simulink model "OPC_linea_transmision_observador"  (R2018a)
settings: Solver=VariableStepAuto  StartTime=0.0  StopTime=inf  RelTol=1e-3
InitFcn:
  | SimulinkInit_linea_transmision
values from neighbouring files (symbols this model uses):
  Ad = sysd.A    [SimulinkInit.m]
  Bd = sysd.B    [SimulinkInit.m]
  Cd = sysd.C    [SimulinkInit.m]
undefined symbols (not defined in the file or in its folder): C1o, C2o, C3o, C4o, F1, F2, F3, F4, H1, H2, H3, H4, K1U, K2U, K3U, K4U, T1, T2, T3, T4, tm
libraries: opclib x12, mpclib x1
settings Model: SimulationMode=accelerator  Creator=cmparedes  LastModifiedBy=MarioAndres

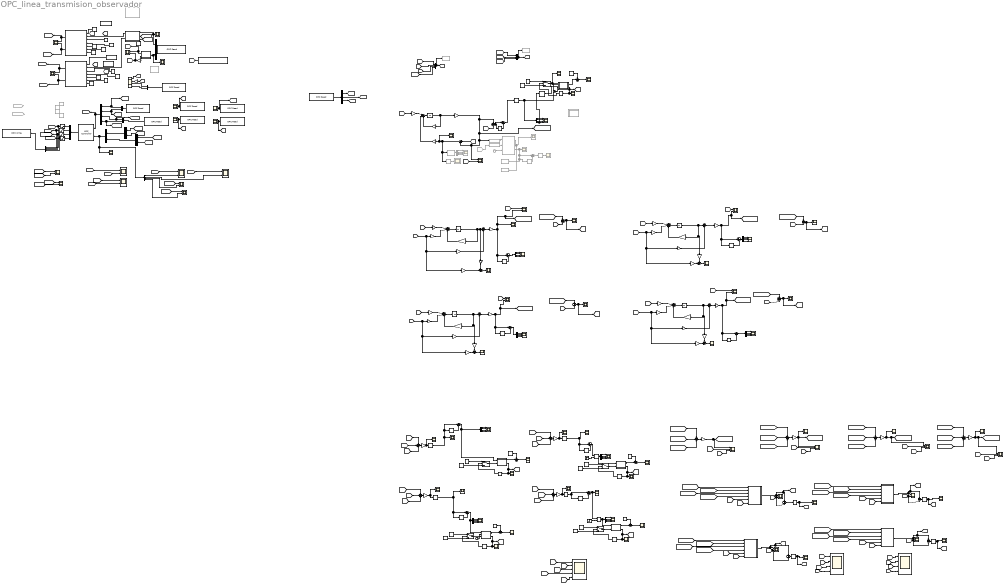
== system OPC_linea_transmision_observador ==
  note: CONTROL TERCIARIO
  note: Attack Quantification
  note: Attack Isolation I2
  note: Attack Isolation I1
  note: Attack Isolation Vsi
  note: Alarm I1
  note: Alarm I3
  note: Alarm I2
  note: Attack Detection
  note: Alarm V
  note: Attack Isolation I3
  Abs{,1..3,5..9} (9 alike) : Abs
  Abs4 : Abs  Commented=on
  Clock : Clock
  Clock1 : Clock  Commented=on
  Clock2 : Clock
  Constant : Constant  Value=2700
  Constant1 : Constant  Commented=on  Value=-13700
  Constant{7..8,10,12,14,22..23,27..28,32} (10 alike) : Constant
  Constant{9,11,21,24,31} (5 alike) : Constant  Value=0
  Constant13 : Constant  Value=500
  Constant15 : Constant  Value=1528
  Constant17 : Constant  Value=1154
  Constant18 : Constant  Value=1000
  Constant2 : Constant  Commented=on  Value=-400
  Constant3 : Constant  Commented=on  Value=5000
  Constant4 : Constant  Commented=on  Value=5000
  Constant5 : Constant  Commented=on  Value=8000
  Constant6 : Constant  Value=115400
  Delay : Delay  DelayLength=1
  Demux{,1..2,4} (4 alike) : Demux  Outputs=2
  Demux{3,5..14} (11 alike) : Demux
  Demux15 : Demux  Outputs=3
  Demux19 : Demux  Commented=on
  Derivative4 : Derivative  Commented=on  CoefficientInTFapproximation=0
  From27 : From  Commented=on  GotoTag=qbio_meas
  From28 : From  Commented=on  GotoTag=pbio_meas
  From60 : From  Commented=on  GotoTag=y_ma
  Gain1 : Gain  Gain=-1
  Gain17 : Gain
  Gain{22..29} (8 alike) : Gain  Gain=1/3
  LinearProg2 : MATLAB Function  TreatAsAtomicUnit=on  SystemSampleTime=1e-3
  LinearProg3 : MATLAB Function  TreatAsAtomicUnit=on  SystemSampleTime=1e-3
  MATLAB Funcionando sin Vload conectado despues del ataque : MATLAB Function  Commented=on  TreatAsAtomicUnit=on
  MATLAB Function : MATLAB Function  TreatAsAtomicUnit=on
  MATLAB Function1 : MATLAB Function  Commented=on  TreatAsAtomicUnit=on
  MATLAB Function12 : MATLAB Function  TreatAsAtomicUnit=on
  MATLAB Function13 : MATLAB Function  TreatAsAtomicUnit=on
  MATLAB Function17 : MATLAB Function  TreatAsAtomicUnit=on
  MATLAB Function18 : MATLAB Function  TreatAsAtomicUnit=on
  MATLAB Function2 : MATLAB Function  TreatAsAtomicUnit=on
  MATLAB Function3 : MATLAB Function  TreatAsAtomicUnit=on
  MATLAB Function34 : MATLAB Function  TreatAsAtomicUnit=on
  MATLAB Function36 : MATLAB Function  TreatAsAtomicUnit=on
  MATLAB Function38 : MATLAB Function  TreatAsAtomicUnit=on
  MATLAB Function39 : MATLAB Function  TreatAsAtomicUnit=on
  MATLAB Function7 : MATLAB Function  Commented=on  TreatAsAtomicUnit=on
  MATLAB Function8 : MATLAB Function  Commented=on  TreatAsAtomicUnit=on
  MPC Controller : mpclib/MPC Controller  SCDEnableBlockLinearizationSpecification=on  mpcobj=mpcobj  is_multiple=0  enable_value=0  return_u0=off  updateMPCinCallerWorkspace=on  ref_from_ws=off  ref_signal_name=[]  ref_preview=off  md_from_ws=off  md_signal_name=[]  md_preview=off  from_project=off  project_file=MPCtask.mat  md_inport=off  mv_inport=off  cost_outport=off  return_sequence=off  return_qpstatus=off  return_state=off  state_inport=off  lims_inport=off  cc_inport=off  ywt_inport=off  is_designfromscratch=0  uwt_inport=off  duwt_inport=off  rhoeps_inport=off  uref_inport=off  n_ts=0.1  n_p=100  n_mv=4  n_md=0  n_ud=0  n_mo=4  n_uo=0  BlockDataType=double  SampleTimeInherited=off  switch_inport=off
  Memory{,1..13} (14 alike) : Memory
  Memory14 : Memory  Commented=on
  Mux : Mux
  Mux3 : Mux  Inputs=2
  Mux4 : Mux
  Mux5 : Mux  Inputs=2
  Mux6 : Mux  Inputs=2
  Mux7 : Mux  Inputs=3
  Mux8 : Mux
  OPC Configuration : opclib/OPC Configuration  opcServers=localhost/Kepware.KEPServerEX.V6/10  errMissingItems=Error  errReadWrite=Warn  errShutdown=Error  errRTViolation=Warn  rtEnable=on  speedup=1  showLatency=off  beingUsed=on
      settings: SourceProductName=OPC Toolbox  SourceProductBaseCode=OT
  OPC Read : opclib/OPC Read  serverHost=localhost  serverID=Kepware.KEPServerEX.V6  itemIDs=Carga_Reno_Channel.Carga.Group1.SOC, Carga_Reno_Channel.Carga.Group1.Lref  readMode=Synchronous (cache)  dataType=double  updateRate=0.1  showQual=off  showTS=off  tsMode=Seconds since start
      settings: SourceProductName=OPC Toolbox  SourceProductBaseCode=OT
  OPC Read1 : opclib/OPC Read  serverHost=localhost  serverID=Kepware.KEPServerEX.V6  itemIDs=Carga_Reno_Channel.Carga.Group1.Vload  readMode=Synchronous (cache)  dataType=double  updateRate=0.1  showQual=off  showTS=off  tsMode=Seconds since start
      settings: SourceProductName=OPC Toolbox  SourceProductBaseCode=OT
  OPC Read2 : opclib/OPC Read  serverHost=localhost  serverID=Kepware.KEPServerEX.V6  itemIDs=Bio_Channel.Bio.Group1.Ibio  readMode=Synchronous (cache)  dataType=double  updateRate=0.1  showQual=off  showTS=off  tsMode=Seconds since start
      settings: SourceProductName=OPC Toolbox  SourceProductBaseCode=OT
  OPC Read3 : opclib/OPC Read  serverHost=localhost  serverID=Kepware.KEPServerEX.V6  itemIDs=Diesel_Channel.Diesel.Group1.Idiesel  readMode=Synchronous (cache)  dataType=double  updateRate=0.1  showQual=off  showTS=off  tsMode=Seconds since start
      settings: SourceProductName=OPC Toolbox  SourceProductBaseCode=OT
  OPC Read4 : opclib/OPC Read  serverHost=localhost  serverID=Kepware.KEPServerEX.V6  itemIDs=Carga_Reno_Channel.Carga.Group1.Pm, Carga_Reno_Channel.Carga.Group1.Qm  readMode=Synchronous (cache)  dataType=double  updateRate=0.1  showQual=off  showTS=off  tsMode=Seconds since start
      settings: SourceProductName=OPC Toolbox  SourceProductBaseCode=OT
  OPC Read5 : opclib/OPC Read  serverHost=localhost  serverID=Kepware.KEPServerEX.V6  itemIDs=Carga_Reno_Channel.Carga.Group1.KB  readMode=Synchronous (cache)  dataType=double  updateRate=0.1  showQual=off  showTS=off  tsMode=Seconds since start
      settings: SourceProductName=OPC Toolbox  SourceProductBaseCode=OT
  OPC Read6 : opclib/OPC Read  serverHost=localhost  serverID=Kepware.KEPServerEX.V6  itemIDs=Carga_Reno_Channel.Carga.Group1.Ipv  readMode=Synchronous (cache)  dataType=double  updateRate=0.1  showQual=off  showTS=off  tsMode=Seconds since start
      settings: SourceProductName=OPC Toolbox  SourceProductBaseCode=OT
  OPC Read7 : opclib/OPC Read  serverHost=localhost  serverID=Kepware.KEPServerEX.V6  itemIDs=Bio_Channel.Bio.Group1.Pm, Bio_Channel.Bio.Group1.Qm  readMode=Synchronous (cache)  dataType=double  updateRate=0.1  showQual=off  showTS=off  tsMode=Seconds since start
      settings: SourceProductName=OPC Toolbox  SourceProductBaseCode=OT
  OPC Read8 : opclib/OPC Read  serverHost=localhost  serverID=Kepware.KEPServerEX.V6  itemIDs=Carga_Reno_Channel.Carga.Group1.Po_reno, Carga_Reno_Channel.Carga.Group1.Qo_reno  readMode=Synchronous (cache)  dataType=double  updateRate=0.1  showQual=off  showTS=off  tsMode=Seconds since start
      settings: SourceProductName=OPC Toolbox  SourceProductBaseCode=OT
  OPC Read9 : opclib/OPC Read  serverHost=localhost  serverID=Kepware.KEPServerEX.V6  itemIDs=Bio_Channel.Bio.Group1.DuC, Carga_Reno_Channel.Carga.Group1.DuC_reno, Diesel_Channel.Diesel.Group1.DieselDutyC  readMode=Synchronous (cache)  dataType=double  updateRate=0.1  showQual=off  showTS=off  tsMode=Seconds since start
      settings: SourceProductName=OPC Toolbox  SourceProductBaseCode=OT
  OPC Write : opclib/OPC Write  serverHost=localhost  serverID=Kepware.KEPServerEX.V6  itemIDs=Bio_Channel.Bio.Group1.Pref, Bio_Channel.Bio.Group1.Qref, Carga_Reno_Channel.Carga.Group1.Pi_reno, Carga_Reno_Channel.Carga.Group1.Qi_reno  writeMode=Synchronous  updateRate=0
      settings: SourceProductName=OPC Toolbox  SourceProductBaseCode=OT
  Pbmax : Constant  Value=1000
  Pbmax1 : Constant  Value=1000
  Pdmax : Constant  Value=1200
  Pdmax1 : Constant  Value=800
  Product2 : Product
  Product4 : Product
  Saturation : Saturate  UpperLimit=12000  LowerLimit=-10000
  Saturation1 : Saturate  UpperLimit=12000  LowerLimit=-10000
  Saturation2 : Saturate  UpperLimit=14000  LowerLimit=-10000
  Saturation3 : Saturate  UpperLimit=10000  LowerLimit=-10000
  Scope{,2..3,7..9,25,30..32,34,41..49,51,55..57,61,64..73,75,110,112,114,118,120..121,135} (43 alike) : Scope
  Scope{1,5..6,10..18,52..53,58,86..89,109} (20 alike) : Scope  NumInputPorts=2
  Scope{59..60,62,138} (4 alike) : Scope  NumInputPorts=3
  Scope{19,36,50,139} (4 alike) : Scope  Commented=on
  Scope{4,33,63,76..83,85} (12 alike) : Scope  NumInputPorts=4
  Scope54 : Scope  Commented=on  NumInputPorts=4
  Scope84 : Scope  NumInputPorts=5
  Signal Specification : SignalSpecification  Commented=on  Dimensions=4
  Signal Specification1 : SignalSpecification  Commented=on  Dimensions=4
  Step13 : Step  Time=0.1  SampleTime=0
  Step14 : Step  Time=0.1  SampleTime=0
  Sum{10,22,38,74} (4 alike) : Sum  Inputs=|++
  Sum{16,18,27,33,42,67,70,72..73} (9 alike) : Sum  Inputs=+-
  Sum{17,20,24..26,30,36..37,39..40} (10 alike) : Sum  Inputs=|+-
  Sum{19,31..32,71} (4 alike) : Sum  Inputs=-+|
  Sum{21,23,49,75..76} (5 alike) : Sum  Inputs=|+++  SampleTime=tm
  Sum{28..29,34..35,53} (5 alike) : Sum  Inputs=+-|
  Sum41 : Sum  Commented=on  Inputs=|+-
  Sum{58..61,77..80} (8 alike) : Sum  Inputs=+++
  Switch{,1..4} (5 alike) : Switch  Criteria=u2 > Threshold
  To Workspace : ToWorkspace  Commented=on  VariableName=det1  SampleTime=1e-4
  To Workspace1 : ToWorkspace  Commented=on  VariableName=norm1  SampleTime=1e-4
  To Workspace2 : ToWorkspace  Commented=on  VariableName=y_ma  SampleTime=1e-4
  To Workspace3 : ToWorkspace  Commented=on  VariableName=u_fs  SampleTime=1e-4
  Unit Delay{1..2,6..7,10} (5 alike) : UnitDelay  SampleTime=tm
  adis1 : Gain  Gain=F3  Multiplication=Matrix(K*u) (u vector)  SampleTime=tm
  adis10 : Gain  Gain=Ld'  Multiplication=Matrix(K*u) (u vector)  SampleTime=tm
  adis11 : Gain  Gain=F1  Multiplication=Matrix(K*u) (u vector)  SampleTime=tm
  adis12 : Gain  Gain=F2  Multiplication=Matrix(K*u) (u vector)  SampleTime=tm
  adis2 : Gain  Gain=F4  Multiplication=Matrix(K*u) (u vector)  SampleTime=tm
  adis7 : Gain  Gain=Ad  Multiplication=Matrix(K*u) (u vector)  SampleTime=tm
  bdis1 : Gain  Gain=T3*Bd  Multiplication=Matrix(K*u) (u vector)  SampleTime=tm
  bdis10 : Gain  Gain=T2*Bd  Multiplication=Matrix(K*u) (u vector)  SampleTime=tm
  bdis11 : Gain  Gain=K2U  Multiplication=Matrix(K*u) (u vector)  SampleTime=tm
  bdis12 : Gain  Gain=H2  Multiplication=Matrix(K*u) (u vector)  SampleTime=tm
  bdis13 : Gain  Gain=eye(1)-C2o*H2  Multiplication=Matrix(K*u) (u vector)  SampleTime=tm
  bdis14 : Gain  Gain=eye(1)-C1o*H1  Multiplication=Matrix(K*u) (u vector)  SampleTime=tm
  bdis15 : Gain  Gain=C1o  Multiplication=Matrix(K*u) (u vector)  SampleTime=tm
  bdis16 : Gain  Gain=C2o  Multiplication=Matrix(K*u) (u vector)  SampleTime=tm
  bdis17 : Gain  Gain=T4*Bd  Multiplication=Matrix(K*u) (u vector)  SampleTime=tm
  bdis18 : Gain  Gain=K4U  Multiplication=Matrix(K*u) (u vector)  SampleTime=tm
  bdis19 : Gain  Gain=H4  Multiplication=Matrix(K*u) (u vector)  SampleTime=tm
  bdis2 : Gain  Gain=K3U  Multiplication=Matrix(K*u) (u vector)  SampleTime=tm
  bdis20 : Gain  Gain=eye(1)-C4o*H4  Multiplication=Matrix(K*u) (u vector)  SampleTime=tm
  bdis21 : Gain  Gain=C4o  Multiplication=Matrix(K*u) (u vector)  SampleTime=tm
  bdis3 : Gain  Gain=H3  Multiplication=Matrix(K*u) (u vector)  SampleTime=tm
  bdis4 : Gain  Gain=eye(1)-C3o*H3  Multiplication=Matrix(K*u) (u vector)  SampleTime=tm
  bdis5 : Gain  Gain=Bd  Multiplication=Matrix(K*u) (u vector)  SampleTime=tm
  bdis6 : Gain  Gain=C3o  Multiplication=Matrix(K*u) (u vector)  SampleTime=tm
  bdis7 : Gain  Gain=T1*Bd  Multiplication=Matrix(K*u) (u vector)  SampleTime=tm
  bdis8 : Gain  Gain=K1U  Multiplication=Matrix(K*u) (u vector)  SampleTime=tm
  bdis9 : Gain  Gain=H1  Multiplication=Matrix(K*u) (u vector)  SampleTime=tm
  cdis{1..5} (5 alike) : Gain  Gain=Cd  Multiplication=Matrix(K*u) (u vector)  SampleTime=tm
  kbP : Constant
  kbQ : Constant
  kdP : Constant
  kdQ : Constant
  wires:
  LinearProg2/1(Pbo) -> [Pbio], Scope16/1
  LinearProg2/2(Pdo) -> [Pdiesel], Scope16/2
  Pdmax1/1 -> LinearProg3/5(QdMax)
  kdP/1 -> LinearProg2/4(kd)
  LinearProg3/2(Qdo) -> Scope15/2, [Qdiesel]
  MATLAB Function2/2(MaxQ) -> LinearProg3/2(Q_e_alt)
  LinearProg3/1(Qbo) -> [Qbio], Scope15/1
  MATLAB Function2/1(MaxP) -> LinearProg2/2(P_e_alt)
  kdQ/1 -> LinearProg3/4(kd)
  Gain17/1 -> Scope1/2, [Q_load]
  OPC Read/1 -> Demux1/1
  Demux1/1 -> MATLAB Function2/1(SOC), Scope2/1
  MATLAB Function/2(Qref) -> Gain17/1
  MATLAB Function/1(Pref) -> Scope1/1, [P_load]
  OPC Read4/1 -> Demux2/1
  Demux2/1 -> Scope4/3
  Demux2/2 -> Scope4/4
  [P_load] -> Scope4/1
  Demux1/2 -> Scope/1, MATLAB Function/1(Lref)
  Gain1/1 -> Scope4/2
  [Q_load] -> Gain1/1
  OPC Read5/1 -> [Kb]
  Constant15/1 -> LinearProg2/1(P_load)
  Pdmax/1 -> LinearProg2/5(PdMax)
  Pbmax/1 -> LinearProg2/6(PbMax)
  Constant18/1 -> LinearProg2/7(P_e_alt_min)
  Pbmax1/1 -> LinearProg3/6(QbMax)
  Constant13/1 -> LinearProg3/7(Q_e_alt_min)
  Demux/2 -> Mux4/2, [Qo_bio]
  Demux3/4 -> Saturation3/1
  MPC Controller/1 -> Demux3/1
  Demux3/3 -> Saturation2/1
  Mux6/1 -> Mux3/2
  Demux4/2 -> [Qo_diesel], Mux4/4
  Demux3/1 -> Saturation/1
  Demux3/2 -> Saturation1/1
  Mux4/1 -> [Paparente], MPC Controller/1
  Demux/1 -> Mux4/1, [Po_bio]
  Mux5/1 -> Mux3/1
  [Pbio] -> Mux5/1
  [Qbio] -> Mux5/2
  [Pdiesel] -> Mux6/1
  [Qdiesel] -> Mux6/2
  [Qo_diesel] -> Scope17/1
  [Qi_bio] -> Scope5/2
  [Po_diesel] -> Scope18/1
  [Pi_Diesel] -> Scope18/2
  [Qi_diesel] -> Scope17/2
  [Pi_bio] -> Scope6/2
  [Qo_bio] -> Scope5/1
  [Po_bio] -> Scope6/1
  OPC Read1/1 -> [V_vsi], Scope3/1
  OPC Read2/1 -> [I1], Scope7/1
  OPC Read3/1 -> [I3], Scope8/1
  OPC Read6/1 -> [I2], Scope9/1
  OPC Read7/1 -> Demux/1
  OPC Read8/1 -> Demux4/1
  Demux4/1 -> [Po_diesel], Mux4/3
  kbP/1 -> LinearProg2/3(kb)
  Constant6/1 -> LinearProg3/1(Q_load)
  [Qo_diesel] -> MATLAB Function2/2(q)
  [Po_diesel] -> MATLAB Function2/3(p)
  kbQ/1 -> LinearProg3/3(kb)
  Saturation/1 -> Mux/1, [Pi_bio]
  Saturation1/1 -> Mux/2, [Qi_bio]
  Saturation2/1 -> Mux/3, [Pi_Diesel]
  Saturation3/1 -> Mux/4, [Qi_diesel]
  Mux/1 -> OPC Write/1
  [Po_diesel] -> Scope11/1
  [Qo_bio] -> Scope12/1
  [Po_bio] -> Scope13/1
  [Qo_diesel] -> Scope10/1
  Mux3/1 -> Demux6/1, Scope32/1, MPC Controller/2
  Demux6/1 -> Scope13/2
  Demux6/2 -> Scope12/2
  Demux6/3 -> Scope11/2
  Demux6/4 -> Scope10/2
  [e2] -> Scope63/2
  Step14/1 -> Product4/2
  Product4/1 -> MATLAB Function18/1(dr), Demux13/1
  Sum77/1 -> Gain22/1
  Clock/1 -> MATLAB Function12/4(t)
  [y_ma] -> Sum70/2
  bdis3/1 -> Sum38/2
  bdis16/1 -> Sum32/1
  [I3] -> Mux8/3
  Sum24/1 -> Demux11/1, MATLAB Function13/1(dr)
  [y_ma] -> Sum17/1
  [x_hat_uio11] -> Sum58/1
  Clock2/1 -> MATLAB Function13/3(t)
  [x_hat_uio21] -> Sum67/1
  Switch/1 -> MATLAB Function36/2(ban)
  Sum35/1 -> Scope51/1
  [y_ma] -> Scope60/3
  Sum10/1 -> cdis1/1
  Demux12/1 -> Scope82/1
  Product2/1 -> MATLAB Function17/1(dr), Demux12/1
  Sum32/1 -> Scope66/1
  Signal Specification1/1 -> MATLAB Function8/2(y_m)
  Sum41/1 -> Abs4/1
  Sum16/1 -> Abs6/1
  Demux5/4 -> Scope77/4
  Sum38/1 -> cdis3/1
  [x_hat_uio1] -> MATLAB Function3/1(x_hat1)
  Constant9/1 -> Switch1/1
  [ca1] -> Scope85/1
  Mux7/1 -> To Workspace3/1, [u_fs]
  Sum73/1 -> [druo3], Scope44/1
  [ca4] -> Scope85/4
  [x_hat] -> Scope60/2
  [V_vsi] -> Mux8/4
  [x_hat_uio11] -> Sum60/1
  [rol] -> MATLAB Function34/6(rol)
  [I2] -> bdis14/1, bdis9/1, bdis8/1
  Abs7/1 -> [e2], Scope70/1
  [x_hat_uio2] -> MATLAB Function34/2(x_hat2)
  Demux9/2 -> Scope79/2
  [y_ma] -> Scope59/3
  Abs8/1 -> [e4], Scope71/1
  [I1] -> Mux8/1
  [y_ma] -> Scope62/3
  [y_ma] -> Scope138/3
  [x_hat] -> Scope138/2
  [a3] -> Sum42/2, Scope58/2
  Switch4/1 -> MATLAB Function13/2(ban)
  Sum61/1 -> Gain27/1
  Sum42/1 -> Abs9/1
  Demux9/4 -> Scope79/4
  Gain24/1 -> Abs1/1, Scope114/1
  Delay/1 -> MATLAB Function12/3(dr1)
  Demux7/3 -> Scope76/3
  Memory6/1 -> Switch2/2
  [ca2] -> Scope85/2
  Sum20/1 -> Demux10/1, MATLAB Function36/1(dr)
  Step13/1 -> Product2/2
  [ruo3] -> Scope84/4
  bdis1/1 -> Sum49/1
  Memory2/1 -> Sum24/2
  Abs1/1 -> Memory2/1, Sum24/1, Scope31/1
  Gain29/1 -> Scope59/1, Scope41/1, [x_hat_uio2]
  Demux13/1 -> Scope83/1
  Constant27/1 -> Switch3/3
  MATLAB Function3/1(v1) -> [ca4], Sum27/1, Scope52/1
  Sum18/1 -> Abs7/1
  Gain22/1 -> Abs/1, Scope110/1
  Abs6/1 -> [e1], Scope64/1
  [e1] -> Scope63/1
  Sum60/1 -> Gain26/1
  [x_hat] -> Scope59/2
  [a4] -> Sum27/2, Scope52/2
  [x_hat_uio12] -> Sum58/2
  Gain27/1 -> Scope135/1, Scope62/1, [x_hat_uio4]
  Sum29/1 -> Scope55/1
  Demux8/1 -> Scope78/1
  [a2] -> Sum18/2, Scope53/2
  [x_hat_uio3] -> MATLAB Function3/3(x_hat3)
  Abs9/1 -> [e3], Scope73/1
  [rol] -> MATLAB Function3/6(rol)
  [ruo4] -> MATLAB Function3/5(ruo1)
  Constant31/1 -> Switch4/1
  [x_hat_uio12] -> Sum59/2
  [x_hat_uio3] -> MATLAB Function34/3(x_hat3)
  Demux9/3 -> Scope79/3
  Gain28/1 -> Scope138/1, [x_hat_uio1]
  Sum37/1 -> Demux5/1
  Gain26/1 -> Scope42/1, Scope60/1, [x_hat_uio3]
  [x_hat] -> Scope62/2
  [x_hat_uio21] -> Sum59/1
  [x_hat_uio13] -> Sum59/3
  [x_hat_uio21] -> Sum60/3
  [x_hat_uio3] -> MATLAB Function38/3(x_hat3)
  [u3] -> Mux7/3
  Memory9/1 -> Switch4/2
  [y_ma] -> Scope88/1
  MATLAB Function39/1(v1) -> [ca3], Sum42/1, Scope58/1
  MATLAB Function8/1(rol) -> To Workspace/1, Scope19/1
  [x_hat_uio4] -> MATLAB Function3/4(x_hat4)
  [ruo2] -> MATLAB Function34/5(ruo1)
  Sum39/1 -> Demux8/1
  [x_hat_uio11] -> Sum61/1
  Demux9/1 -> Scope79/1
  [e4] -> Scope63/4
  bdis4/1 -> Sum71/2
  [x_hat_uio4] -> MATLAB Function34/4(x_hat4)
  [druo2] -> Sum78/1
  [ruo2] -> Scope84/3
  Sum36/1 -> Demux7/1
  [ruo1] -> MATLAB Function38/5(ruo1)
  [x_hat_uio1] -> MATLAB Function39/1(x_hat1)
  [x_hat_uio13] -> Sum58/3
  Constant32/1 -> Switch4/3
  Demux13/3 -> Scope83/3
  [x_hat_uio4] -> MATLAB Function39/4(x_hat4)
  bdis18/1 -> Sum76/2
  Demux5/2 -> Scope77/2
  Demux13/4 -> Scope83/4
  cdis3/1 -> Memory12/1, Sum39/1, Scope88/2, [x_hat_uio13]
  [u_fs] -> bdis5/1
  Abs4/1 -> Scope36/1
  Memory14/1 -> Sum41/2
  bdis11/1 -> Sum23/2
  [rol] -> MATLAB Function39/6(rol)
  [druo1] -> Sum77/1
  Abs5/1 -> Demux14/1, MATLAB Function12/1(dr)
  Demux14/2 -> Scope33/2
  Demux14/3 -> Scope33/3
  Demux12/3 -> Scope82/3
  Constant22/1 -> Switch2/3
  Demux12/4 -> Scope82/4
  Demux12/2 -> Scope82/2
  Demux11/3 -> Scope81/3
  [x_hat_uio2] -> MATLAB Function38/2(x_hat2)
  Demux11/1 -> Scope81/1
  Demux10/3 -> Scope80/3
  Demux10/4 -> Scope80/4
  Demux10/1 -> Scope80/1
  [x_hat_uio2] -> MATLAB Function3/2(x_hat2)
  Abs2/1 -> Memory3/1, Sum25/1, Scope34/1
  Demux14/1 -> Scope33/1
  Sum33/1 -> Sum30/1, Memory7/1
  Demux14/4 -> Delay/1, Scope33/4
  Sum25/1 -> Product2/1
  Sum17/1 -> Derivative4/1, MATLAB Function7/1(r), Scope48/1, adis10/1
  Demux8/3 -> Scope78/3
  Demux8/2 -> Scope78/2
  [x_hat_uio4] -> MATLAB Function38/4(x_hat4)
  Demux7/2 -> Scope76/2
  Demux5/3 -> Scope77/3
  [x_hat_uio3] -> MATLAB Function39/3(x_hat3)
  [x_hat_uio11] -> Sum70/1
  Switch1/1 -> MATLAB Function17/2(ban)
  Demux5/1 -> Scope77/1
  [u1] -> Mux7/1
  Demux11/2 -> Scope81/2
  Abs/1 -> Memory/1, Sum20/1, Scope25/1
  Memory13/1 -> Sum40/2
  Memory7/1 -> Sum30/2
  Memory11/1 -> Sum37/2
  [x_hat_uio1] -> MATLAB Function38/1(x_hat1)
  [a1] -> Sum16/2, Scope109/2
  Memory10/1 -> Sum36/2
  Sum79/1 -> Gain24/1
  Constant28/1 -> Sum35/1
  Sum75/1 -> Unit Delay6/1
  Unit Delay2/1 -> bdis21/1, adis2/1, Sum74/1
  bdis2/1 -> Sum49/2
  Demux8/4 -> Scope78/4
  Sum30/1 -> Abs5/1
  MATLAB Function12/1(r) -> Sum34/2
  Sum34/1 -> Scope68/1
  [u2] -> Mux7/2
  [ruo3] -> MATLAB Function39/5(ruo1)
  Memory8/1 -> Switch3/2
  MATLAB Function34/1(v1) -> [ca2], Sum18/1, Scope53/1
  Switch3/1 -> Scope75/1, MATLAB Function12/2(ban)
  Constant23/1 -> Sum34/1
  MATLAB Function18/1(r) -> Sum29/2
  Memory12/1 -> Sum39/2
  Constant21/1 -> Switch2/1
  [x_hat_uio2] -> MATLAB Function39/2(x_hat2)
  [druo3] -> Sum77/3
  Memory/1 -> Sum20/2
  MATLAB Function17/2(c) -> [ruo2], Scope49/1, Memory5/1
  MATLAB Function13/1(r) -> Sum35/2
  [x_hat_uio1] -> MATLAB Function34/1(x_hat1)
  MATLAB Function13/2(c) -> [ruo3], Scope57/1, Memory9/1
  [I1] -> bdis20/1, bdis19/1, bdis18/1
  Constant11/1 -> Switch/1
  [druo2] -> Sum77/2
  Constant10/1 -> Switch1/3
  Constant8/1 -> Sum28/1
  Memory4/1 -> Sum26/2
  Memory3/1 -> Sum25/2
  Constant7/1 -> Sum53/1
  MATLAB Function12/2(c) -> [rol], Scope69/1, Memory8/1
  [ca3] -> Scope85/3
  Memory1/1 -> Switch/2
  Sum53/1 -> Scope120/1
  bdis6/1 -> Sum71/1
  MATLAB Function36/2(c) -> [ruo1], Scope121/1, Memory1/1
  [y_ma] -> Sum33/2
  Sum78/1 -> Gain23/1
  MATLAB Function38/1(v1) -> [ca1], Sum16/1, Scope109/1
  Sum72/1 -> [druo2], Scope43/1
  MATLAB Function17/1(r) -> Sum28/2
  Constant12/1 -> Sum29/1
  [x_hat_uio21] -> Sum61/2
  [x_hat_uio13] -> Sum60/2
  [ruo4] -> Scope84/5
  Gain25/1 -> Scope118/1, Abs3/1
  Sum26/1 -> Product4/1, Scope46/1
  Constant24/1 -> Switch3/1
  Demux7/4 -> Scope76/4
  Gain23/1 -> Abs2/1, Scope112/1
  MATLAB Function18/2(c) -> [ruo4], Scope56/1, Memory6/1
  [rol] -> MATLAB Function38/6(rol)
  [druo2] -> Sum80/2
  Sum80/1 -> Gain25/1
  [druo1] -> Sum79/2
  adis7/1 -> Sum75/3
  [x_hat_uio12] -> Sum61/3
  [druo4] -> Sum78/3
  [druo3] -> Sum78/2
  [x_hat_uio13] -> Sum73/1
  [y_ma] -> Sum72/2
  Sum67/1 -> [druo4], Scope45/1
  [x_hat_uio12] -> Sum72/1
  [y_ma] -> Sum67/2
  bdis8/1 -> Sum21/2
  Demux19/1 -> Scope54/1
  Sum58/1 -> Gain28/1
  Demux13/2 -> Scope83/2
  Sum70/1 -> [druo1], Scope30/1
  Sum28/1 -> Scope47/1
  Sum27/1 -> Abs8/1
  [e3] -> Scope63/3
  cdis1/1 -> Memory10/1, Sum36/1, [x_hat_uio11], Scope86/2, Scope61/1
  [druo3] -> Sum79/1
  Constant14/1 -> Switch/3
  [druo1] -> Sum80/3
  Switch2/1 -> MATLAB Function18/2(ban)
  [druo4] -> Sum80/1
  cdis2/1 -> Memory11/1, Sum37/1, Scope87/2, [x_hat_uio12]
  Demux10/2 -> Scope80/2
  Sum71/1 -> Scope67/1
  Memory5/1 -> Switch1/2
  Sum74/1 -> cdis5/1
  Sum31/1 -> Scope65/1
  bdis19/1 -> Sum74/2
  Sum22/1 -> cdis2/1
  [y_ma] -> Scope87/1
  adis2/1 -> Sum76/3
  [u_fs] -> bdis1/1
  bdis20/1 -> Sum19/2
  Sum19/1 -> Scope72/1
  cdis4/1 -> Sum33/1, [x_hat], Signal Specification/1, Scope14/1, Sum17/2
  bdis7/1 -> Sum21/1
  [druo4] -> Sum79/3
  Sum23/1 -> Unit Delay10/1
  bdis17/1 -> Sum76/1
  adis1/1 -> Sum49/3
  Demux7/1 -> Scope76/1
  [I3] -> bdis13/1, bdis12/1, bdis11/1
  Sum21/1 -> Unit Delay7/1
  adis10/1 -> Sum75/2
  Sum40/1 -> Demux9/1
  Demux11/4 -> Scope81/4
  bdis14/1 -> Sum31/2
  Abs3/1 -> Memory4/1, Sum26/1
  Unit Delay1/1 -> bdis6/1, adis1/1, Sum38/1
  Sum76/1 -> Unit Delay2/1
  adis11/1 -> Sum21/3
  Demux19/2 -> Scope54/2
  Unit Delay6/1 -> cdis4/1, adis7/1
  [u_fs] -> bdis10/1
  adis12/1 -> Sum23/3
  bdis10/1 -> Sum23/1
  MATLAB Function36/1(r) -> Sum53/2
  [u_fs] -> bdis7/1
  Demux19/3 -> Scope54/3
  Sum59/1 -> Gain29/1
  [y_ma] -> Scope14/2
  Demux19/4 -> Scope54/4
  [y_ma] -> Scope86/1
  Clock1/1 -> MATLAB Function8/3(tiempo)
  From60/1 -> Signal Specification1/1
  bdis13/1 -> Sum32/2
  cdis5/1 -> Memory13/1, Sum40/1, [x_hat_uio21], Scope89/2
  Derivative4/1 -> Scope139/1
  Mux8/1 -> To Workspace2/1, [y_ma]
  Sum49/1 -> Unit Delay1/1
  bdis9/1 -> Sum10/2
  [rol] -> Scope84/1
  Unit Delay7/1 -> adis11/1, bdis15/1, Sum10/1
  [I2] -> Mux8/2
  bdis12/1 -> Sum22/2
  bdis5/1 -> Sum75/1
  [y_ma] -> Scope89/1
  MATLAB Function8/2(norm_rd) -> Sum41/1, Memory14/1, To Workspace1/1, Scope50/1
  bdis21/1 -> Sum19/1
  [u_fs] -> bdis17/1
  MATLAB Function7/1(y) -> Demux19/1
  bdis15/1 -> Sum31/1
  [ruo1] -> Scope84/2
  Unit Delay10/1 -> bdis16/1, adis12/1, Sum22/1
  [y_ma] -> Sum73/2
  [V_vsi] -> bdis4/1, bdis3/1, bdis2/1
  Signal Specification/1 -> MATLAB Function8/1(y_hat)
  OPC Read9/1 -> Demux15/1
  Demux15/1 -> [u1]
  Demux15/2 -> [u2]
  Demux15/3 -> [u3]

== matlab function OPC_linea_transmision_observador/MATLAB Function ==
  data: Lref input; Pref output; Qref output
function [Pref,Qref] = fcn(Lref)

Pref = 1000;
Qref = 1000;%sqrt(Lref^2 - Pref^2);

== matlab function OPC_linea_transmision_observador/MATLAB Function3 ==
  data: x_hat1 input; v1 output; x_hat2 input; x_hat3 input; x_hat4 input; ruo1 input; rol input
function v1 = fcn(x_hat1,x_hat2,x_hat3,x_hat4,ruo1,rol)

% yol=[u1 ; u2];
% ym=[ym1 ; ym2];
%  C1=[zeros(1,10) 1];
 C1=[0 0 0 1];
 v11=C1*(x_hat4-x_hat1)*ruo1*rol;
 v12=C1*(x_hat4-x_hat2)*ruo1*rol;
 v13=C1*(x_hat4-x_hat3)*ruo1*rol;
 
 v1=-(v11+v12+v13);

== matlab function OPC_linea_transmision_observador/LinearProg2 ==
  data: P_load input; Pbo output; P_e_alt input; kb input; kd input; PdMax input; PbMax input; Pdo output; P_e_alt_min input
function [Pbo, Pdo] = fcn(P_load, P_e_alt, kb, kd, PdMax, PbMax, P_e_alt_min)

% P_load es la potencia que se requiere en la carga.

% P_e_alt es la potencia estimada de generacion de las energias
% alternativas

% kb y kd son los pesos de las funcion de costo.

% las salidas son las potencias optimas para bio y diesel

Pb=0;
Pd=0;

D_P_e_alt = P_e_alt - P_e_alt_min; % superaavit de energia alternativa.

flagDelt = 0;

if(D_P_e_alt >= P_load)
    flagDelt = 1;
end
   

if(flagDelt==0)
    P_trad = P_load - D_P_e_alt;
    % flag: variable que indica si tiene sentido evaluar los
    % if's que se encuentran mas adelante. es decir, si flag = 0 
    % despues del primer if entonces NO se le esta pidiendo al sistema
    % mas potencia de la que puede generar y portanto el problema de 
    % optimizacion lineal tiene sentido.
    % entonces 
    flag=0;

    if(P_trad>PdMax+PbMax)
        Pd=PdMax;
        Pb=PbMax;
        flag=1;
    end

    % si ambas energias tienen el mismo factor de costo.
    if(kd==kb && flag==0)
        Pb=P_trad/2;
        Pd=P_trad/2;
    end

    % si la energia diesel es mas cara que la biomasa.
    if(kd>kb && flag==0)
        if(P_trad<=PbMax)
            Pb=P_trad;
            Pd=0;
        else
            Pb=PbMax;
            Pd=P_trad-PbMax;
        end
    end

    % si la biomasa es mas cara que la diesel.
    if(kd<kb && flag==0)
        if(P_trad<=PdMax)
            Pd=P_trad;
            Pb=0;
        else
            Pd=PdMax;
            Pb=P_trad-PdMax;
        end
    end
end

Pbo=Pb;
Pdo=Pd;

== matlab function OPC_linea_transmision_observador/LinearProg3 ==
  data: Q_load input; Qbo output; Q_e_alt input; kb input; kd input; QdMax input; QbMax input; Qdo output; Q_e_alt_min input
function [Qbo, Qdo] = fcn(Q_load, Q_e_alt, kb, kd, QdMax, QbMax, Q_e_alt_min)

% Q_load es la Qotencia que se requiere en la carga.

% Q_e_alt es la Qotencia estimada de generacion de las energias
% alternativas

% kb y kd son los Qesos de las funcion de costo.

% las salidas son las Qotencias oQtimas Qara bio y diesel

Qb=0;
Qd=0;

D_Q_e_alt = Q_e_alt - Q_e_alt_min; % suQeraavit de energia alternativa.

flagDelt = 0;

if(D_Q_e_alt >= Q_load)
    flagDelt = 1;
end
   

if(flagDelt==0)
    Q_trad = Q_load - D_Q_e_alt;
    % flag: variable que indica si tiene sentido evaluar los
    % if's que se encuentran mas adelante. es decir, si flag = 0 
    % desQues del Qrimer if entonces NO se le esta Qidiendo al sistema
    % mas Qotencia de la que Quede generar y Qortanto el Qroblema de 
    % oQtimizacion lineal tiene sentido.
    % entonces 
    flag=0;

    if(Q_trad>QdMax+QbMax)
        Qd=QdMax;
        Qb=QbMax;
        flag=1;
    end

    % si ambas energias tienen el mismo factor de costo.
    if(kd==kb && flag==0)
        Qb=Q_trad/2;
        Qd=Q_trad/2;
    end

    % si la energia diesel es mas cara que la biomasa.
    if(kd>kb && flag==0)
        if(Q_trad<=QbMax)
            Qb=Q_trad;
            Qd=0;
        else
            Qb=QbMax;
            Qd=Q_trad-QbMax;
        end
    end

    % si la biomasa es mas cara que la diesel.
    if(kd<kb && flag==0)
        if(Q_trad<=QdMax)
            Qd=Q_trad;
            Qb=0;
        else
            Qd=QdMax;
            Qb=Q_trad-QdMax;
        end
    end
end

Qbo=Qb;
Qdo=Qd;

== matlab function OPC_linea_transmision_observador/MATLAB Function2 ==
  data: SOC input; MaxP output; MaxQ output; q input; p input
function [MaxP, MaxQ] = fcn(SOC,q,p)


%  funcion que calcula la potencia maxima que puede suministrar las fuentes
%  renovables deacuerdo a la cantidad de carga que hay almancenada en la
%  bateria. esta va de 0 a 100%


% estoc valores que aparecen a continuacion se pusieron de manera
% arbitraria. corresponde a una persona con especialidad en la parte de
% potencia electrica determinar el verdadero algoritmo para hallar la
% potencia que deberia suministrar el nodo de energia renovable deacuerdo a
% la carga de la bateria.

MaxP = 0;
MaxQ = 0;

if( SOC >= 90 )
    MaxP = p;
    MaxQ = q;
end

if( SOC <= 90 )
    MaxP = 0.9*p;
    MaxQ = 0.9*q;
end

if( SOC <= 70 )
    MaxP = 0.7*p;
    MaxQ = 0.7*q;
end

if( SOC <= 60 )
    MaxP = 0.4*p;
    MaxQ = 0.4*q;
end

== matlab function OPC_linea_transmision_observador/MATLAB Funcionando sin Vload conectado despues del ataque ==
  data: dr input; r output; ban input; c output
function [r,c]   = fcn(dr,ban)



th1=20; %para i1, i2 y v
th2=10;
th3=50;
th4=2;%2; (para vsi)  %1 (otro)
if ban==1
    r=1;
    c=0;
    %     if abs(dr(1))>th || abs(dr(2))>th || abs(dr(4))>th
    if dr(2)>th2 || dr(4)>th4 || dr(1)>th1 || dr(3)>th3
        c=1;
        r=0;
    end
else
    r=0;
    c=1;
%     if abs(dr(1))>th || abs(dr(2))>th || abs(dr(4))>th %%&& ban==0
    if dr(2)>th2 || dr(4)>th4 || dr(1)>th1 || dr(3)>th3 %%&& ban==0
        c=0;
        r=1;
    end
end

% ra=r;
% a=0;

== matlab function OPC_linea_transmision_observador/MATLAB Function1 ==
  data: SOC input; MaxP output; MaxQ output
function [MaxP, MaxQ] = fcn(SOC)


%  funcion que calcula la potencia maxima que puede suministrar las fuentes
%  renovables deacuerdo a la cantidad de carga que hay almancenada en la
%  bateria. esta va de 0 a 100%


% estoc valores que aparecen a continuacion se pusieron de manera
% arbitraria. corresponde a una persona con especialidad en la parte de
% potencia electrica determinar el verdadero algoritmo para hallar la
% potencia que deberia suministrar el nodo de energia renovable deacuerdo a
% la carga de la bateria.

MaxP = 0;
MaxQ = 0;

if( SOC >= 90 )
    MaxP = 500;
    MaxQ = 5000;
end

if( SOC <= 90 )
    MaxP = 200;
    MaxQ = 4000;
end

if( SOC <= 70 )
    MaxP = 100;
    MaxQ = 1000;
end

if( SOC <= 60 )
    MaxP = 50;
    MaxQ = 500;
end

== matlab function OPC_linea_transmision_observador/MATLAB Function12 ==
  data: dr input; r output; ban input; c output; dr1 input; t input
function [r,c]   = fcn(dr,ban,dr1,t)


m=dr(4)-dr1;
th1=1;%1;%20; %para i1, i2 y v
if t>1
    th1=2;
end
th2=2;%1;%10;
th3=50;
th4=0.2;%1;%2; (para vsi)  %1 (otro)
if ban==1
    r=1;
    c=0;
    %     if abs(dr(1))>th || abs(dr(2))>th || abs(dr(4))>th
    if dr(2)>th2 || (dr(4)>th4 && m>0) || dr(1)>th1 || dr(3)>th3
        c=1;
        r=0;
    end
else
    r=0;
    c=1;
%     if abs(dr(1))>th || abs(dr(2))>th || abs(dr(4))>th %%&& ban==0
    if dr(2)>th2 || ( dr(4)>th4 && m>0)|| dr(1)>th1 || dr(3)>th3 %%&& ban==0
        c=0;
        r=1;
    end
end

% ra=r;
% a=0;

== matlab function OPC_linea_transmision_observador/MATLAB Function13 ==
  data: dr input; r output; ban input; c output; t input
function [r,c]   = fcn(dr,ban,t)

% if t<=0.33
%     th=1.5e4;
%     %     v=2;
% elseif t<=0.55
%     th=2e4;
%     %     v=3;
% else
%     th=3e3;
% end

% r=0;
% c=1;

th=10;
to1=1;%2;
to2=1;%5;
to4=0.2;%0.4;

if ban==1
    r=1;
    c=0;
    if abs(dr(3))>th && abs(dr(1))<to1 && abs(dr(2))<to2 && abs(dr(4))<to4 && t>0.12
        c=1;
        r=0;
    end
else
    r=0;
    c=1;
    if abs(dr(3))>th && abs(dr(1))<to1 && abs(dr(2))<to2 && abs(dr(4))<to4 && t>0.12%%&& ban==0
        c=0;
        r=1;
    end
end

% ra=r;
% a=0;

== matlab function OPC_linea_transmision_observador/MATLAB Function17 ==
  data: dr input; r output; ban input; c output
function [r,c]   = fcn(dr,ban)

% if t<=0.33
%     th=1.5e4;
%     %     v=2;
% elseif t<=0.55
%     th=2e4;
%     %     v=3;
% else
%     th=3e3;
% end

% r=0;
% c=1;

th=2;%8; % 5 antiguamente
to1=0.5;%2;
to3=21;
to4=0.2;

if ban==1
    r=1;
    c=0;
    if abs(dr(2))>th && abs(dr(1))<to1 && abs(dr(3))<to3 && abs(dr(4))<to4
        c=1;
        r=0;
    end
else
    r=0;
    c=1;
    if abs(dr(2))>th && abs(dr(1))<2 && abs(dr(3))<to3 && abs(dr(4))<to4 %%&& ban==0
        c=0;
        r=1;
    end
end

% ra=r;
% a=0;

== matlab function OPC_linea_transmision_observador/MATLAB Function18 ==
  data: dr input; r output; ban input; c output
function [r,c]   = fcn(dr,ban)

% if t<=0.33
%     th=1.5e4;
%     %     v=2;
% elseif t<=0.55
%     th=2e4;
%     %     v=3;
% else
%     th=3e3;
% end

% r=0;
% c=1;

th=0.2;%0.52;
to1=1;%2;
to2=1;%5;
to3=21;

if ban==1
    r=1;
    c=0;
    if abs(dr(4))>th && abs(dr(1))<to1 && abs(dr(2))< to2 && abs(dr(3))<to3
        c=1;
        r=0;
    end
else
    r=0;
    c=1;
    if abs(dr(4))>th && abs(dr(1))<to1 && abs(dr(2))< to2 && abs(dr(3))<to3%%&& ban==0
        c=0;
        r=1;
    end
end

% ra=r;
% a=0;

== matlab function OPC_linea_transmision_observador/MATLAB Function7 ==
  data: r input; y output
function y = fcn(r)%u1,u2,ym1,ym2)

r1=r(1)/2000;%200;
r2=r(2)/2000;%500;
r3=r(3)/2000;%1300;
r4=r(4)/2000;
y=[r1 r2 r3 r4];
% if norm_rd >=Th_det
%     rol=1;
% else
%     rol=0;
% end

== matlab function OPC_linea_transmision_observador/MATLAB Function8 ==
  data: y_hat input; rol output; y_m input; norm_rd output; tiempo input
function [rol,norm_rd] = fcn(y_hat,y_m,tiempo)%u1,u2,ym1,ym2)
% Th_det = 6.5e-8;
Th_det=0.2;%2.3e-2; %Funciona bien si los pulsos no estan tan separados

if tiempo <=0.12 || (tiempo>=2.88 && tiempo<=2.92)
    Th_det=8;
end
% Th_det=38;
% yol=[u1 ; u2];
% ym=[ym1 ; ym2];

rd1=y_hat(1)-y_m(1)
rd2=y_hat(2)-y_m(2)
rd3=y_hat(3)-y_m(3) 
rd4=y_hat(4)-y_m(4)

% rd=y_hat-y_m;
rd=[rd1 rd2 rd3 rd4];
norm_rd=sqrt(sum(rd.^2));
if tiempo <0.12
    norm_rd=0;
end
% sys=tf(1,[0.001 1]);


if norm_rd >=Th_det && tiempo>=0.12%Th_det_up && norm_rd <=Th_det_down
    rol=1;
else
    rol=0;
end

== matlab function OPC_linea_transmision_observador/MATLAB Function34 ==
  data: x_hat1 input; v1 output; x_hat2 input; x_hat3 input; x_hat4 input; ruo1 input; rol input
function v1 = fcn(x_hat1,x_hat2,x_hat3,x_hat4,ruo1,rol)

% yol=[u1 ; u2];
% ym=[ym1 ; ym2];
%  C1=[zeros(1,4) 1 zeros(1,6)];
 C1=[0 1 0 0];
 v11=C1*(x_hat2-x_hat1)*ruo1*rol;
 v12=C1*(x_hat2-x_hat3)*ruo1*rol;
 v13=C1*(x_hat2-x_hat4)*ruo1*rol;
 
 v1=-(v11+v12+v13);

== matlab function OPC_linea_transmision_observador/MATLAB Function38 ==
  data: x_hat1 input; v1 output; x_hat2 input; x_hat3 input; x_hat4 input; ruo1 input; rol input
function v1 = fcn(x_hat1,x_hat2,x_hat3,x_hat4,ruo1,rol)

% yol=[u1 ; u2];
% ym=[ym1 ; ym2];
%  C1=[zeros(1,3) 1 zeros(1,7)]; 
 C1=[1 zeros(1,3)]; 
 v11=C1*(x_hat1-x_hat2)*ruo1*rol;
 v12=C1*(x_hat1-x_hat3)*ruo1*rol;
 v13=C1*(x_hat1-x_hat4)*ruo1*rol;
 
 v1=-(v11+v12+v13);

== matlab function OPC_linea_transmision_observador/MATLAB Function36 ==
  data: dr input; r output; ban input; c output
function [r,c]   = fcn(dr,ban)

% if t<=0.33
%     th=1.5e4;
%     %     v=2;
% elseif t<=0.55
%     th=2e4;
%     %     v=3;
% else
%     th=3e3;
% end

% r=0;
% c=1;

th=1.9;%5;
to2=1;%3;
to3=21;
to4=0.1;%0.4;

if ban==1
    r=1;
    c=0;
    if abs(dr(1))>th && abs(dr(2))<to2 && abs(dr(3))<to3 && abs(dr(4))<to4
        c=1;
        r=0;
    end
else
    r=0;
    c=1;
    if abs(dr(1))>th && abs(dr(2))<to2 && abs(dr(3))<to3 && abs(dr(4))<to4%%&& ban==0
        c=0;
        r=1;
    end
end

% ra=r;
% a=0;

== matlab function OPC_linea_transmision_observador/MATLAB Function39 ==
  data: x_hat1 input; v1 output; x_hat2 input; x_hat3 input; x_hat4 input; ruo1 input; rol input
function v1 = fcn(x_hat1,x_hat2,x_hat3,x_hat4,ruo1,rol)

% yol=[u1 ; u2];
% ym=[ym1 ; ym2];
%  C1=[zeros(1,5) 1 zeros(1,5)]; 
 C1=[0 0 1 0];
 v11=C1*(x_hat3-x_hat1)*ruo1*rol;
 v12=C1*(x_hat3-x_hat2)*ruo1*rol;
 v13=C1*(x_hat3-x_hat4)*ruo1*rol;
 
 v1=-(v11+v12+v13);
